simulink model "w1p1"  (R2020b)
settings: Solver=VariableStepAuto  StartTime=0.0  StopTime=10.0  MaxStep=0.01  RelTol=1e-3
model workspace (MAT data in the model file):
  K1 = 50
  K12 = 80
  M1 = 100
  M2 = 95
  b = 50
settings Model: Creator=family  LastModifiedBy=family

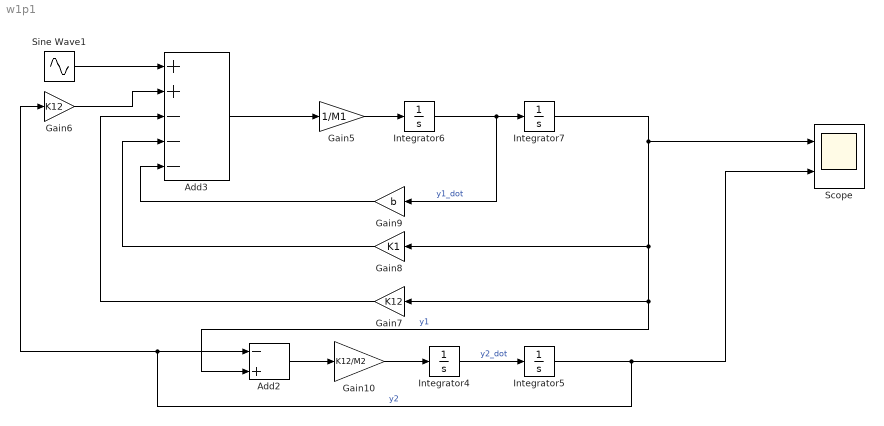
== system w1p1 ==
  Add2 : Sum  Inputs=-+
  Add3 : Sum  Inputs=++---
  Gain10 : Gain  Gain=K12/M2
  Gain5 : Gain  Gain=1/M1
  Gain6 : Gain  Gain=K12
  Gain7 : Gain  Gain=K12
  Gain8 : Gain  Gain=K1
  Gain9 : Gain  Gain=b
  Integrator{4..7} (4 alike) : Integrator
  Scope : Scope  NumInputPorts=2
  Sine Wave1 : Sin  Amplitude=3  Frequency=10  SampleTime=0
  wires:
  Integrator7/1 -> Scope/1, Add2/2, Gain7/1, Gain8/1  "y1"
  Gain9/1 -> Add3/5
  Gain5/1 -> Integrator6/1
  Gain10/1 -> Integrator4/1
  Gain7/1 -> Add3/3
  Integrator5/1 -> Scope/2, Add2/1, Gain6/1  "y2"
  Integrator4/1 -> Integrator5/1  "y2_dot"
  Sine Wave1/1 -> Add3/1
  Add2/1 -> Gain10/1
  Gain6/1 -> Add3/2
  Gain8/1 -> Add3/4
  Add3/1 -> Gain5/1
  Integrator6/1 -> Gain9/1, Integrator7/1  "y1_dot"
